simulink model "Copy_of_modello_completo_2_12"  (R2020b)
settings: Solver=FixedStepDiscrete  StartTime=0.0  StopTime=Inf  FixedStep=0.02  RelTol=1e-3  EnableMultiTasking=on
undefined symbols (not defined in the file or in its folder): attuatore_Amax, attuatore_Amin, attuatore_Emax, attuatore_Emin, attuatore_Rmax, attuatore_Rmin, attuatore_Tmax, attuatore_Tmin, DiscIntNeverNeededParam, interventoA_05, interventoA_1, interventoE_05, interventoE_1, interventoT, inv_A, inv_comp_h, inv_E, inv_R, inv_T, K_AW_B_AP_quota, K_AW_B_becc, K_AW_B_imb, K_AW_B_roll, K_imb_inv, Kd_h_app, Kd_h_flare, Ki_AP_quota_select, Ki_AP_rotta, Ki_AP_vel, Ki_becch, Ki_h_app, Ki_h_cruise, Ki_h_flare, Ki_roll, Kp_AP_quota_hold_h, Kp_AP_quota_hold_l, Kp_AP_quota_select, Kp_AP_rotta, Kp_AP_vel, Kp_becch, Kp_comp_h, Kp_h_app_max, Kp_h_app_min, Kp_h_cruise, Kp_h_flare, Kp_imb, Kp_p, Kp_q, Kp_roll, Kp_Rotta_ATO, Newton, phi_max, phi_min, Raphson, safe_phi, safe_V, t_AP, theta_max, theta_min, time_alarm_SAFE ... (+5)
libraries: simulink_extras x41, arduinolib x26, pid_lib x8, svdutilitieslib x6, simulink x3, dspsigops x3, aerolibtransform2sys x2, aerolibtransform2 x2, cstblocks x1
(part 7 of 8)

== matlab function Copy_of_modello_completo_2_12/AUTOPILOTA/Subsystem1/Subsystem1/ALLINEAMENTO ==
  data: modo input; lat input; long input; h input; psi input; WP_db_info input; WP_db_param input; e_h output; vel output; lat_comandato output; long_comandato output; distance output; QUOTA output; ROTTA output; counter input; counter_out output
function [e_h,vel,lat_comandato,long_comandato,distance,QUOTA,ROTTA,counter_out] = autoland(modo,lat,long,h,psi,WP_db_info,WP_db_param,counter)
%#codegen
%WP_db_info=(nWP_tot n_WP frame command current autocontinue)
%per Nav
%WP_db_param=(velocità, autocontinue, vuoto, vuoto, lat_comandato, long_comandato, h_comandato)

persistent flag 

if isempty (flag)
    flag = 0;
end

%Definizione posizione waypoints
lat_comandato = WP_db_param(counter,5);
long_comandato = WP_db_param(counter,6);
h_comandato = WP_db_param(counter,7);

e_h = h_comandato - h; %errore quota

%Calcolo distanza velivolo-waypoint inseguito
a = (sin(((lat_comandato-lat)*pi/180)/2))^2+cos(lat*pi/180)*cos(lat_comandato*pi/180)*(sin(((long_comandato-long)*pi/180)/2))^2;
c = 2*atan2(sqrt(a),sqrt(1-a));
distance = 6378137*c;               

%Calcolo distanza velivolo-waypoint precedente
if counter > 1
    psi_ref = atan2(sin((WP_db_param(counter,6)-WP_db_param(counter-1,6))*pi/180)*cos(WP_db_param(counter,5)*pi/180),cos(WP_db_param(counter-1,5)*pi/180)*sin(WP_db_param(counter,5)*pi/180)-sin(WP_db_param(counter-1,5)*pi/180)*cos(WP_db_param(counter,5)*pi/180)*cos((WP_db_param(counter,6)-WP_db_param(counter-1,6))*pi/180))*180/pi;     %psi di riferimento
    a_pre = (sin(((lat-WP_db_param(counter-1,5))*pi/180)/2))^2+cos(WP_db_param(counter-1,5)*pi/180)*cos(lat*pi/180)*(sin(((long-WP_db_param(counter-1,6))*pi/180)/2))^2;
    c_pre = 2*atan2(sqrt(a_pre),sqrt(1-a_pre));
    dist = 6378137*c_pre;                                                  %distanza velivolo-WP precedente
else
    psi_ref = atan2(sin((long_comandato-long)*pi/180)*cos(lat_comandato*pi/180),cos(lat*pi/180)*sin(lat_comandato*pi/180)-sin(lat*pi/180)*cos(lat_comandato*pi/180)*cos((long_comandato-long)*pi/180))*180/pi;
    dist = 0;
end

if psi_ref < 0
    psi_ref = 360 - abs(psi_ref);
end

autocontinue=WP_db_param(counter,2); 

%Definizione angolo tra WP successivi
if autocontinue == 1
    a_fut = (sin(((WP_db_param(counter+1,5)-WP_db_param(counter,5))*pi/180)/2))^2+cos(WP_db_param(counter,5)*pi/180)*cos(WP_db_param(counter+1,5)*pi/180)*(sin(((WP_db_param(counter+1,6)-WP_db_param(counter,6))*pi/180)/2))^2;
    c_fut = 2*atan2(sqrt(a_fut),sqrt(1-a_fut));
    dist_fut = 6378137*c_fut;    %distanza waypoint inseguito - waypoint successivo
    psi_ref_fut = atan2(sin((WP_db_param(counter+1,6)-WP_db_param(counter,6))*pi/180)*cos(WP_db_param(counter+1,5)*pi/180),cos(WP_db_param(counter,5)*pi/180)*sin(WP_db_param(counter+1,5)*pi/180)-sin(WP_db_param(counter,5)*pi/180)*cos(WP_db_param(counter+1,5)*pi/180)*cos((WP_db_param(counter+1,6)-WP_db_param(counter,6))*pi/180))*180/pi;      %distanza WP-WP+1
    if psi_ref_fut < 0
        psi_ref_fut = 360 - abs(psi_ref_fut);
    end
    if counter > 1
        angoloWP = abs(psi_ref_fut - psi_ref);
    else 
        angoloWP = abs(psi_ref_fut - (atan2(sin((long_comandato-long)*pi/180)*cos(lat_comandato*pi/180),cos(lat*pi/180)*sin(lat_comandato*pi/180)-sin(lat*pi/180)*cos(lat_comandato*pi/180)*cos((long_comandato-long)*pi/180))*180/pi));
    end
else
    dist_fut = 0;
    angoloWP = 0;
end


if counter < 2
    angoloWP_pre = 0;
elseif counter == 2
    angoloWP_pre = abs(psi_ref - atan2(sin((WP_db_param(counter-1,6)-long)*pi/180)*cos(WP_db_param(counter-1,5)*pi/180),cos(lat*pi/180)*sin(WP_db_param(counter-1,5)*pi/180)-sin(lat*pi/180)*cos(WP_db_param(counter-1,5)*pi/180)*cos((WP_db_param(counter-1,6)-long)*pi/180))*180/pi);
else
    psi_ref_pre = atan2(sin((WP_db_param(counter-1,6)-WP_db_param(counter-2,6))*pi/180)*cos(WP_db_param(counter-1,5)*pi/180),cos(WP_db_param(counter-2,5)*pi/180)*sin(WP_db_param(counter-1,5)*pi/180)-sin(WP_db_param(counter-2,5)*pi/180)*cos(WP_db_param(counter-1,5)*pi/180)*cos((WP_db_param(counter-1,6)-WP_db_param(counter-2,6))*pi/180))*180/pi;
if psi_ref_pre < 0
    psi_ref_pre = 360 - abs(psi_ref_pre);
end
    angoloWP_pre = abs(psi_ref - psi_ref_pre);
end
    
if angoloWP <=3                                  % Condizione aggiunta da Sensolini, altrimenti l'errore in atterraggio era troppo grande
    error = 1;
    tolleranza_distWP_fut = 20;
elseif angoloWP <= 10
    error = 30;                                       %Definizione raggio di errore 
    tolleranza_distWP_fut = 100;                      %Definizione distanza minima accettabile tra WP successivi
elseif angoloWP > 10 && angoloWP <= 50 
    error = 80;
    tolleranza_distWP_fut = 250;
elseif angoloWP > 50 && angoloWP <= 90     
    error = 100;
    tolleranza_distWP_fut = 300;
elseif angoloWP > 90 && angoloWP <= 120     
    error = 150;
    tolleranza_distWP_fut = 350;
else     
    error = 200;
    tolleranza_distWP_fut = 400;
end

nWP=size(WP_db_param,1);

%Definizione distanza dal WP precedente per correzione traiettoria

if angoloWP_pre <= 10
    soglia_dist = 80;                                   
elseif angoloWP_pre > 10 && angoloWP_pre <= 50 
    soglia_dist = 200;
elseif angoloWP_pre > 50 && angoloWP_pre <= 90 
    soglia_dist = 300;
elseif angoloWP_pre > 90 && angoloWP_pre <= 120 
    soglia_dist = 350;
else
    soglia_dist = 400;
end

k=1.3;    %fattore moltiplicativo correzione rotta

%Definizione rotta
if autocontinue == 1  
    
    psi_comandato = atan2(sin((long_comandato - long)*pi/180)*cos(lat_comandato*pi/180),cos(lat*pi/180)*sin(lat_comandato*pi/180)-sin(lat*pi/180)*cos(lat_comandato*pi/180)*cos((long_comandato - long)*pi/180))*180/pi;     %rotta da seguire
    vel = WP_db_param(counter,1);                   %velocità di approccio al wp
    psi_comandato_fut = atan2(sin((WP_db_param(counter+1,6)-long)*pi/180)*cos(WP_db_param(counter+1,5)*pi/180),cos(lat*pi/180)*sin(WP_db_param(counter+1,5)*pi/180)-sin(lat*pi/180)*cos(WP_db_param(counter+1,5)*pi/180)*cos((WP_db_param(counter+1,6)-long)*pi/180))*180/pi;
    
    if vel <= 20                                    %Definizione raggio di errore in base alla velocità di volo
        error = error*1.1;
    elseif (vel <= 25 && vel > 20)
        error = error*1.2;
    elseif (vel <= 30 && vel > 25)
        error = error*1.3;
    else 
        error = error*1.4;
    end
    
        if dist < soglia_dist && distance > error
            psi_comandato = atan2(sin((long_comandato - long)*pi/180)*cos(lat_comandato*pi/180),cos(lat*pi/180)*sin(lat_comandato*pi/180)-sin(lat*pi/180)*cos(lat_comandato*pi/180)*cos((long_comandato - long)*pi/180))*180/pi;
        elseif dist > soglia_dist && distance > error
            psi_comandato = atan2(sin((long_comandato - long)*pi/180)*cos(lat_comandato*pi/180),cos(lat*pi/180)*sin(lat_comandato*pi/180)-sin(lat*pi/180)*cos(lat_comandato*pi/180)*cos((long_comandato - long)*pi/180))*180/pi;
            err = abs ( psi_comandato - psi_ref );             %errore inseguimento rotta
            if (psi_ref <= 90 && psi_ref >= 0)                 %primo quadrante
                if psi_comandato > psi_ref
                    psi_comandato = psi_comandato + k*err;
                elseif psi_comandato < psi_ref
                    psi_comandato = psi_comandato - k*err;
                else
                    psi_comandato = psi_comandato;
                end                   
            elseif (psi_ref <= 180 && psi_ref > 90)             %quarto quadrante
                if psi_ref*psi_comandato > 0
                    if psi_comandato > psi_ref || ( psi_comandato < -90 && psi_comandato > -180)
                        psi_comandato = psi_comandato + k*err;
                    elseif psi_comandato < psi_ref
                        psi_comandato = psi_comandato - k*err;
                    else
                        psi_comandato = psi_comandato;
                    end                      
                else
                    err = abs ( 360 - abs(psi_comandato) - psi_ref); 
                    if psi_comandato > psi_ref || ( psi_comandato < -90 && psi_comandato > -180)
                        psi_comandato = psi_comandato + k*err;
                    elseif psi_comandato < psi_ref
                        psi_comandato = psi_comandato - k*err;
                    else
                        psi_comandato = psi_comandato;
                    end                     
                end
            elseif(psi_ref < -90 && psi_ref >= -180)             %terzo quadrante
                if psi_ref*psi_comandato > 0
                    if psi_comandato > psi_ref
                        psi_comandato = psi_comandato + k*err;
                    elseif psi_comandato < psi_ref  || (psi_comandato < 180 && psi_comandato > 90)
                        psi_comandato = psi_comandato - k*err;
                    else
                        psi_comandato = psi_comandato;
                    end  
                else
                    err = abs ( 360 -(psi_comandato) - abs(psi_ref)); 
                    if psi_comandato > psi_ref
                        psi_comandato = psi_comandato + k*err;
                    elseif psi_comandato < psi_ref || (psi_comandato < 180 && psi_comandato > 90)
                        psi_comandato = psi_comandato - k*err;
                    else
                        psi_comandato = psi_comandato;
                    end                     
                end
            elseif(psi_ref < 0 && psi_ref >= -90)             %secondo quadrante
                if psi_comandato > psi_ref
                    psi_comandato = psi_comandato + k*err;
                elseif psi_comandato < psi_ref
                    psi_comandato = psi_comandato - k*err;
                else
                    psi_comandato = psi_comandato;
                end
            end
            
        elseif distance < error
            if dist_fut > tolleranza_distWP_fut
                psi_comandato = psi_comandato_fut;
                counter = counter + 1;
            else
                if counter < nWP-1
                    counter = counter + 2;
                else
                    vel=22;
                    h_comandato=h+0.4;
                    psi_comandato=psi+36.6;   
                    e_h=0;
                    flag=1;
                end
            end
        end
         
    
else
    
    psi_comandato = atan2(sin((long_comandato - long)*pi/180)*cos(lat_comandato*pi/180),cos(lat*pi/180)*sin(lat_comandato*pi/180)-sin(lat*pi/180)*cos(lat_comandato*pi/180)*cos((long_comandato - long)*pi/180))*180/pi;
    vel = WP_db_param(counter,1);                   
    error = 40;
    
        if dist < soglia_dist && flag == 0
                  psi_comandato = atan2(sin((long_comandato - long)*pi/180)*cos(lat_comandato*pi/180),cos(lat*pi/180)*sin(lat_comandato*pi/180)-sin(lat*pi/180)*cos(lat_comandato*pi/180)*cos((long_comandato - long)*pi/180))*180/pi;
        elseif dist > soglia_dist && distance > error && flag == 0
                err = abs ( psi_comandato - psi_ref );        
                if (psi_ref <= 90 && psi_ref >= 0)                 %primo quadrante
                    if psi_comandato > psi_ref
                        psi_comandato = psi_comandato + k*err;
                    elseif psi_comandato < psi_ref
                        psi_comandato = psi_comandato - k*err;
                    else
                        psi_comandato = psi_comandato;
                    end 
                elseif (psi_ref <= 180 && psi_ref > 90)             %quarto quadrante
                    if psi_ref*psi_comandato > 0
                        if psi_comandato > psi_ref || ( psi_comandato < -90 && psi_comandato > -180)
                            psi_comandato = psi_comandato + k*err;
                        elseif psi_comandato < psi_ref
                            psi_comandato = psi_comandato - k*err;
                        else
                            psi_comandato = psi_comandato;
                        end
                    else
                        err = abs ( 360 - abs(psi_comandato) - psi_ref); 
                        if psi_comandato > psi_ref || ( psi_comandato < -90 && psi_comandato > -180)
                            psi_comandato = psi_comandato + k*err;
                        elseif psi_comandato < psi_ref
                            psi_comandato = psi_comandato - k*err;
                        else
                            psi_comandato = psi_comandato;
                        end                     
                    end
                elseif(psi_ref < -90 && psi_ref >= -180)             %terzo quadrante
                    if psi_ref*psi_comandato > 0
                        if psi_comandato > psi_ref
                            psi_comandato = psi_comandato + k*err;
                        elseif psi_comandato < psi_ref  || (psi_comandato < 180 && psi_comandato > 90)
                            psi_comandato = psi_comandato - k*err;
                        else
                            psi_comandato = psi_comandato;
                        end 
                    else
                        err = abs ( 360 -(psi_comandato) - abs(psi_ref)); 
                        if psi_comandato > psi_ref
                            psi_comandato = psi_comandato + k*err;
                        elseif psi_comandato < psi_ref || (psi_comandato < 180 && psi_comandato > 90)
                            psi_comandato = psi_comandato - k*err;
                        else
                            psi_comandato = psi_comandato;
                        end                         
                    end
                elseif(psi_ref < 0 && psi_ref >= -90)             %secondo quadrante
                    if psi_comandato > psi_ref
                        psi_comandato = psi_comandato + k*err;
                    elseif psi_comandato < psi_ref
                        psi_comandato = psi_comandato - k*err;
                    else
                        psi_comandato = psi_comandato;
                    end
                end
                
        else            
                vel=22;
                h_comandato=h+0.4;
                psi_comandato=psi+36.6;   
                e_h=0;
                flag=1;                       %con flag=1 l'aereo rimane in loiter senza uscire dal ciclo            
        end
          
end


%se ho nWPtotali=0 (lat,long,alt==0), traiettoria circolare
if lat_comandato == 0 && long_comandato == 0 && h_comandato==0    
    h_comandato=h+0.3;
    psi_comandato=psi+36.6;   
    vel=22;
    e_h=0;   
end

%output  
QUOTA = h_comandato;
ROTTA = psi_comandato;


%se arrivo all'ultimo WP, loiter 
if counter == size(WP_db_param,1) && autocontinue > 0    
    autocontinue = 0;     
end

%I waipoint si resettano una volta conclusa la manovra
if modo == 4
    counter_out = counter;
else
    counter_out = 1;    
end

== matlab function Copy_of_modello_completo_2_12/AUTOPILOTA/Subsystem1/Subsystem1/FLARE/MATLAB Function ==
  data: WP_db_param input; rotta output; lat input; long input
function rotta  = rotta(WP_db_param,lat,long)
%#codegen

lat_comandato = WP_db_param(3,5);      
long_comandato = WP_db_param(3,6);


psi_ref = atan2(sin((WP_db_param(3,6)-WP_db_param(2,6))*pi/180)*cos(WP_db_param(3,5)*pi/180),cos(WP_db_param(2,5)*pi/180)*sin(WP_db_param(3,5)*pi/180)-sin(WP_db_param(2,5)*pi/180)*cos(WP_db_param(3,5)*pi/180)*cos((WP_db_param(3,6)-WP_db_param(2,6))*pi/180))*180/pi;     %psi di riferimento

psi_comandato = atan2(sin((long_comandato - long)*pi/180)*cos(lat_comandato*pi/180),cos(lat*pi/180)*sin(lat_comandato*pi/180)-sin(lat*pi/180)*cos(lat_comandato*pi/180)*cos((long_comandato - long)*pi/180))*180/pi;
err = abs ( psi_comandato - psi_ref ); 
k = 1.4;

if (psi_ref <= 90 && psi_ref >= 0)                 %primo quadrante
                    if psi_comandato > psi_ref
                        psi_comandato = psi_comandato + k*err;
                    elseif psi_comandato < psi_ref
                        psi_comandato = psi_comandato - k*err;
                    else
                        psi_comandato = psi_comandato;
                    end
elseif (psi_ref <= 180 && psi_ref > 90)             %quarto quadrante
                    if psi_ref*psi_comandato > 0
                        if psi_comandato > psi_ref || ( psi_comandato < -90 && psi_comandato > -180)
                            psi_comandato = psi_comandato + k*err;
                        elseif psi_comandato < psi_ref
                            psi_comandato = psi_comandato - k*err;
                        else
                            psi_comandato = psi_comandato;
                        end                      
                    else
                        err = abs ( 360 - abs(psi_comandato) - psi_ref); 
                        if psi_comandato > psi_ref || ( psi_comandato < -90 && psi_comandato > -180)
                            psi_comandato = psi_comandato + k*err;
                        elseif psi_comandato < psi_ref
                            psi_comandato = psi_comandato - k*err;
                        else
                            psi_comandato = psi_comandato;
                        end                     
                    end
elseif(psi_ref < -90 && psi_ref >= -180)             %terzo quadrante
                    if psi_ref*psi_comandato > 0
                        if psi_comandato > psi_ref
                            psi_comandato = psi_comandato + k*err;
                        elseif psi_comandato < psi_ref  || (psi_comandato < 180 && psi_comandato > 90)
                            psi_comandato = psi_comandato - k*err;
                        else
                            psi_comandato = psi_comandato;
                        end  
                    else
                        err = abs ( 360 -(psi_comandato) - abs(psi_ref)); 
                        if psi_comandato > psi_ref
                            psi_comandato = psi_comandato + k*err;
                        elseif psi_comandato < psi_ref || (psi_comandato < 180 && psi_comandato > 90)
                            psi_comandato = psi_comandato - k*err;
                        else
                            psi_comandato = psi_comandato;
                        end                     
                    end
elseif(psi_ref < 0 && psi_ref >= -90)             %secondo quadrante
                    if psi_comandato > psi_ref
                        psi_comandato = psi_comandato + k*err;
                    elseif psi_comandato < psi_ref
                        psi_comandato = psi_comandato - k*err;
                    else
                        psi_comandato = psi_comandato;
                    end
end

rotta = psi_comandato;

== matlab function Copy_of_modello_completo_2_12/AIR RX/MATLAB Function2 ==
  data: mess_out output; Len output; status input; mess_1 input; mess_2 input; buff_prev input; buffer output
function [mess_out,Len,buffer] = fcn(status,mess_1,mess_2,buff_prev)


mess_out=uint8(zeros(1,100));
buffer = uint8(zeros(3,100));
counter = uint8(0);
Len = int32(0);



mess_out = buff_prev(3,:);       %il messaggio in uscita è l'ultima riga
Len = int32(mess_out(1,2));



buffer(1,:) = uint8(zeros(1,100)); %buffer è buff_prev traslato in basso di 1 riga, quindi elimino mess_out
for j=2:1:3
buffer(j,:) = buff_prev(j-1,:);
end
i=3;
while i >= 1                        %cerco la prima riga nulla dal basso
    if buffer(i,:) == 0
        counter = uint8(i);
        break
    end
    i = i-1;
end


if status == 1                   
    buffer(counter,:) = mess_1;
    
elseif status == 2
    buffer(counter,:) = mess_1;
    buffer(counter-1,:) = mess_2;
    
    
else
    buffer(counter,:) = uint8(zeros(1,100));


end



end

== matlab function Copy_of_modello_completo_2_12/AUTOPILOTA/Subsystem1/Subsystem1/CREAZIONE_WAYPOINT /AUTOLANDING_WAYPOINTS ==
  data: WP_info output; WP_param output; Lat_Home input; Long_Home input; h_Home input; alt input; vel_wp1_al input; vel_wp2_al input

function [WP_info,WP_param]  = fcn(Lat_Home,Long_Home,h_Home,alt,vel_wp1_al,vel_wp2_al)
%#codegen

WP_info=zeros(3,6);
WP_param=zeros(3,7);


for i=1:3

    WP_info(i,1)=3;                 %
    WP_info(i,2)=i-1;               % numero del waypoint da 1 a 6
    WP_info(i,3)=16;                % commande del tipo del command
    WP_info(i,4)=0;                 % sistema di riferimento
    WP_info(i,5)=0;                 % current waypoint
    WP_info(i,6)=1;                 %
    
    
    
    
WP_param(i,1)=vel_wp2_al;               %Velocita del WP
WP_param(i,2)=1;                % Autocontinue 1
WP_param(i,3)=0;                % Parametro  non utilizzato
WP_param(i,4)=0;                % Parametro  non utilizzato
WP_param(i,5)=Lat_Home(i);      % LAT
WP_param(i,6)=Long_Home(i);     % LONG
WP_param(i,7)=h_Home+alt(i);    % ALT
    
    
end

WP_param(1,1)=vel_wp1_al;
WP_param(3,2)=0;                % Autocontinue 1

end

== matlab function Copy_of_modello_completo_2_12/AUTOPILOTA/Subsystem1/Subsystem3/GO_HOME ==
  data: lat input; V_goHome output; long input; h input; psi input; Lat_Home input; Long_Home input; h_goHome_rif input; V_goHome_rif input; h_goHome output; RC_goHome output; rotta_goHome output
function [V_goHome, h_goHome, RC_goHome, rotta_goHome] = go_home(lat, long, h, psi, Lat_Home, Long_Home, h_goHome_rif, V_goHome_rif)

persistent flag
if isempty (flag)
    flag = 0;
end

lat_comandato = Lat_Home;
long_comandato = Long_Home;

a = (sin(((lat_comandato-lat)*pi/180)/2))^2+cos(lat*pi/180)*cos(lat_comandato*pi/180)*(sin(((long_comandato-long)*pi/180)/2))^2;
c = 2*atan2(sqrt(a),sqrt(1-a));
distance = 6378137*c; 

rotta_goHome = atan2(sin((long_comandato - long)*pi/180)*cos(lat_comandato*pi/180),cos(lat*pi/180)*sin(lat_comandato*pi/180)-sin(lat*pi/180)*cos(lat_comandato*pi/180)*cos((long_comandato - long)*pi/180))*180/pi;     %rotta da seguire
h_goHome = h_goHome_rif;
V_goHome = V_goHome_rif;
RC_goHome = h_goHome - h;

    if distance < 30 && flag == 0
        flag = 1;
        V_goHome = V_goHome_rif;
        h_goHome = h_goHome_rif + 0.4;
        rotta_goHome = psi + 100;
        RC_goHome = 0;
    end
end

== matlab function Copy_of_modello_completo_2_12/AIR RX/MATLAB Function3 ==
  data: mess_out input; new_mex output; mess_out_prev input
function new_mex = fcn(mess_out,mess_out_prev)
persistent counter

if isempty(counter)
    counter = uint16(0);
end

new_mex = uint16(0);


if ( mess_out(3) ~= mess_out_prev(3) && (all(mess_out ~= 0) == false) )

    if counter > 100
        counter = uint16(0);
    end
    counter = counter +1;
end
new_mex = counter;

end
